simulink model "suspension_r2019a"  (R2019a)
settings: Solver=VariableStepAuto  StartTime=0.0  StopTime=10.0  RelTol=1e-3
InitFcn:
  | M1=320
  | M2=40
  | K1=18000
  | B=1000
  | K2=2e5
settings Model: Creator=byronmason  LastModifiedBy=byronmason
settings DataIOCC: Refine=10

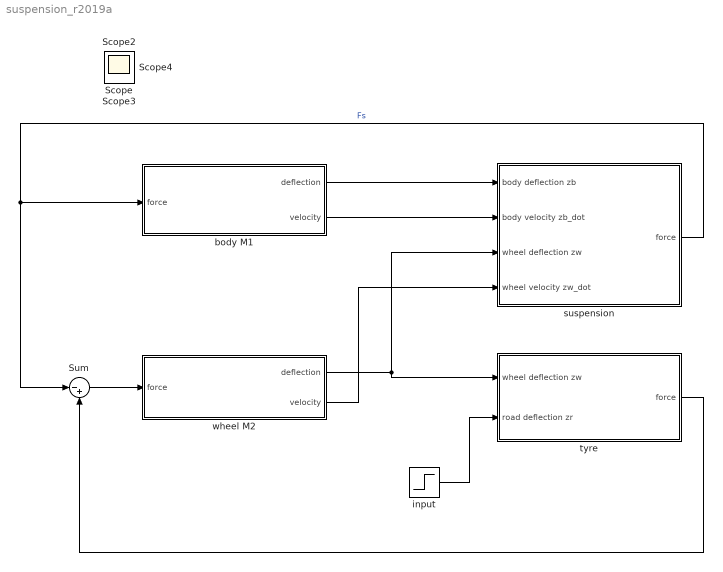
== system suspension_r2019a ==
  Sum : Sum  Inputs=|-+
  body M1 : Subsystem
  input : Step  Time=2  After=0.05  SampleTime=0
  suspension : Subsystem
  tyre : Subsystem
  wheel M2 : Subsystem
  Scope{,2..4} (4 alike) : Scope
  wires:
  body M1/1(deflection) -> suspension/1(body deflection zb)
  body M1/2(velocity) -> suspension/2(body velocity zb_dot)
  suspension/1(force) -> body M1/1(force), Sum/1  "Fs"
  wheel M2/2(velocity) -> suspension/4(wheel velocity zw_dot)
  wheel M2/1(deflection) -> tyre/1(wheel deflection zw), suspension/3(wheel deflection zw)
  tyre/1(force) -> Sum/2
  Sum/1 -> wheel M2/1(force)
  input/1 -> tyre/2(road deflection zr)

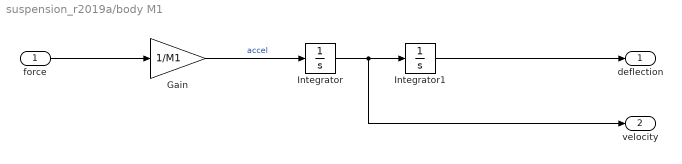
== system suspension_r2019a/body M1 ==
  force : Inport
  Gain : Gain  Gain=1/M1
  Integrator : Integrator
  Integrator1 : Integrator
  deflection : Outport
  velocity : Outport  Port=2
  wires:
  force/1 -> Gain/1
  Integrator/1 -> velocity/1, Integrator1/1
  Integrator1/1 -> deflection/1
  Gain/1 -> Integrator/1  "accel"

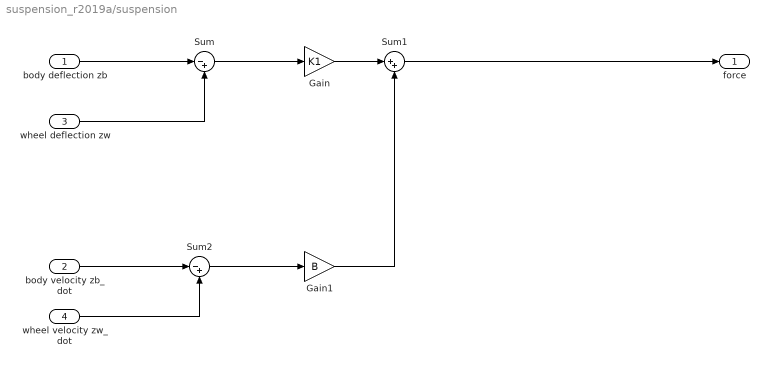
== system suspension_r2019a/suspension ==
  body deflection zb : Inport
  body velocity zb_dot : Inport  Port=2
  wheel deflection zw : Inport  Port=3
  wheel velocity zw_dot : Inport  Port=4
  Gain : Gain  Gain=K1
  Gain1 : Gain  Gain=B
  Sum : Sum  Inputs=|-+
  Sum1 : Sum  Inputs=|++
  Sum2 : Sum  Inputs=|-+
  force : Outport
  wires:
  body deflection zb/1 -> Sum/1
  wheel deflection zw/1 -> Sum/2
  Sum/1 -> Gain/1
  Gain/1 -> Sum1/1
  body velocity zb_dot/1 -> Sum2/1
  wheel velocity zw_dot/1 -> Sum2/2
  Sum2/1 -> Gain1/1
  Gain1/1 -> Sum1/2
  Sum1/1 -> force/1

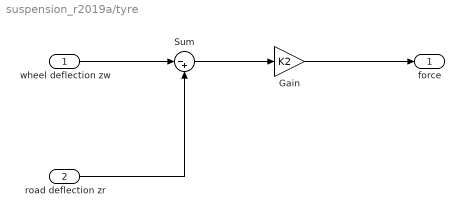
== system suspension_r2019a/tyre ==
  wheel deflection zw : Inport
  road deflection zr : Inport  Port=2
  Gain : Gain  Gain=K2
  Sum : Sum  Inputs=|-+
  force : Outport
  wires:
  wheel deflection zw/1 -> Sum/1
  road deflection zr/1 -> Sum/2
  Sum/1 -> Gain/1
  Gain/1 -> force/1

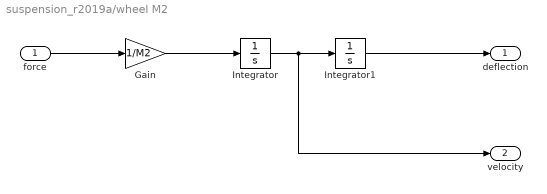
== system suspension_r2019a/wheel M2 ==
  force : Inport
  Gain : Gain  Gain=1/M2
  Integrator : Integrator
  Integrator1 : Integrator
  deflection : Outport
  velocity : Outport  Port=2
  wires:
  force/1 -> Gain/1
  Gain/1 -> Integrator/1
  Integrator/1 -> velocity/1, Integrator1/1
  Integrator1/1 -> deflection/1
